simulink model "Day07"  (R2024b)
settings: Solver=VariableStepAuto  StartTime=0.0  StopTime=10.0  RelTol=1e-3
libraries: simulink x1
settings Model: Creator=jun_mac  LastModifiedBy=jun_mac

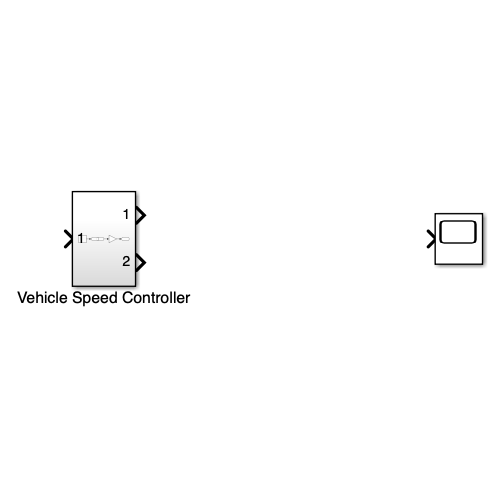
[thumbnail: Simulink's stored preview of the top-level diagram]
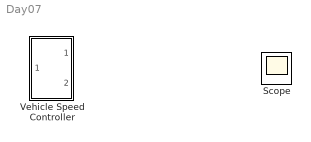
== system Day07 ==
  Scope : Scope
  Vehicle Speed Controller : Subsystem

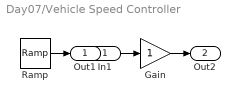
== system Day07/Vehicle Speed Controller ==
  In1 : Inport
  Gain : Gain
  Ramp : simulink/Sources/Ramp  slope=1  start=0  InitialOutput=0
  Out1 : Outport
  Out2 : Outport  Port=2
  wires:
  In1/1 -> Gain/1
  Gain/1 -> Out2/1
  Ramp/1 -> Out1/1
